simulink model "coif1_7_Level"  (R2021a)
settings: Solver=VariableStepAuto  StartTime=0.0  StopTime=8  RelTol=1e-3
undefined symbols (not defined in the file): lambda2
libraries: dspsigops x15, dspquant2 x1
(part 1 of 4)
settings Model: Creator=Bhea Vasquez  LastModifiedBy=Bhea Vasquez

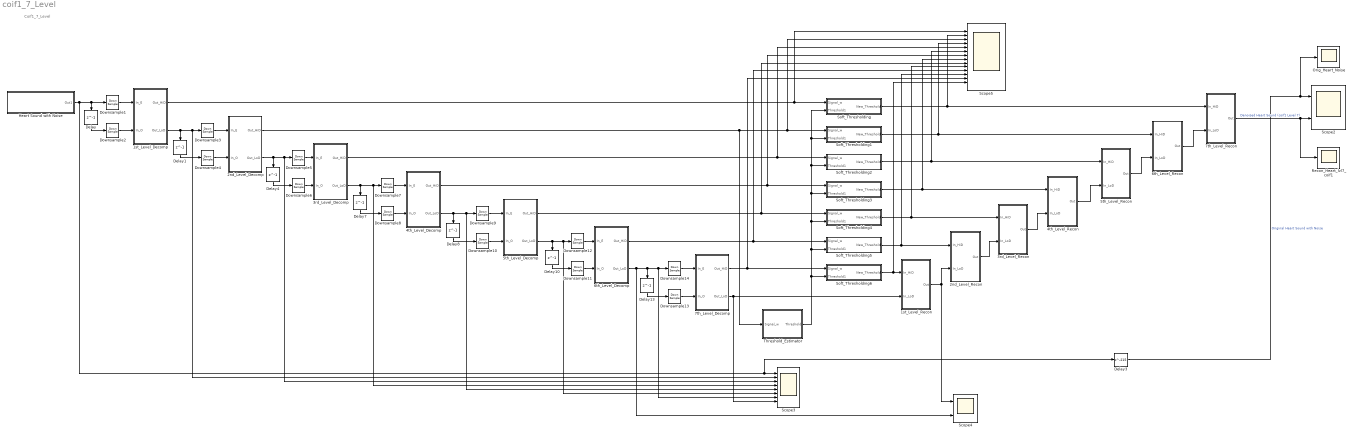
== system coif1_7_Level ==
  note: Coif1_7_Level
  1st_Level_Decomp : Subsystem
  1st_Level_Recon : Subsystem
  2nd_Level_Decomp : Subsystem
  2nd_Level_Recon : Subsystem
  3rd_Level_Decomp : Subsystem
  3rd_Level_Recon : Subsystem
  4th_Level_Decomp : Subsystem
  4th_Level_Recon : Subsystem
  5th_Level_Decomp : Subsystem
  5th_Level_Recon : Subsystem
  6th_Level_Decomp : Subsystem
  6th_Level_Recon : Subsystem
  7th_Level_Decomp : Subsystem
  7th_Level_Recon : Subsystem
  Delay{,1,4,7..8,10,13} (7 alike) : Delay  DelayLength=1  SampleTime=1/44100
  Delay3 : Delay  DelayLength=215  SampleTime=1/44100
  Downsample{1..14} (14 alike) : DownSample  N=30
  Heart Sound with Noise : Subsystem
  Orig_Heart_Noise : Scope
  Recon_Heart_lvl7_coif1 : Scope
  Scope2 : Scope  NumInputPorts=2
  Scope3 : Scope  NumInputPorts=8
  Scope4 : Scope  NumInputPorts=2
  Scope5 : Scope  NumInputPorts=14
  Soft_Thresholding : Subsystem
  Soft_Thresholding1 : Subsystem
  Soft_Thresholding2 : Subsystem
  Soft_Thresholding3 : Subsystem
  Soft_Thresholding4 : Subsystem
  Soft_Thresholding5 : Subsystem
  Soft_Thresholding6 : Subsystem
  Threshold_Estimator : Subsystem
  wires:
  5th_Level_Decomp/2(Out_LoD) -> Scope3/6, Downsample12/1, Delay10/1
  Downsample11/1 -> 6th_Level_Decomp/2(In_O)
  Delay10/1 -> Downsample11/1
  Downsample12/1 -> 6th_Level_Decomp/1(In_E)
  4th_Level_Decomp/2(Out_LoD) -> Scope3/5, Downsample9/1, Delay8/1
  Delay4/1 -> Downsample6/1
  1st_Level_Decomp/2(Out_LoD) -> Scope3/2, Downsample3/1, Delay1/1
  Downsample9/1 -> 5th_Level_Decomp/1(In_E)
  Downsample3/1 -> 2nd_Level_Decomp/1(In_E)
  Heart Sound with Noise/1(Out1) -> Delay3/1, Scope3/1, Downsample1/1, Delay/1
  Downsample6/1 -> 3rd_Level_Decomp/2(In_O)
  Delay7/1 -> Downsample8/1
  Downsample8/1 -> 4th_Level_Decomp/2(In_O)
  Downsample1/1 -> 1st_Level_Decomp/1(In_E)
  Downsample5/1 -> 3rd_Level_Decomp/1(In_E)
  Delay8/1 -> Downsample10/1
  Downsample7/1 -> 4th_Level_Decomp/1(In_E)
  Downsample4/1 -> 2nd_Level_Decomp/2(In_O)
  Delay1/1 -> Downsample4/1
  2nd_Level_Decomp/2(Out_LoD) -> Scope3/3, Downsample5/1, Delay4/1
  Downsample2/1 -> 1st_Level_Decomp/2(In_O)
  3rd_Level_Decomp/2(Out_LoD) -> Scope3/4, Downsample7/1, Delay7/1
  Downsample10/1 -> 5th_Level_Decomp/2(In_O)
  Downsample13/1 -> 7th_Level_Decomp/2(In_O)
  Downsample14/1 -> 7th_Level_Decomp/1(In_E)
  Delay13/1 -> Downsample13/1
  6th_Level_Decomp/2(Out_LoD) -> Scope4/2, Scope3/7, Downsample14/1, Delay13/1
  Threshold_Estimator/1(Threshold) -> Soft_Thresholding6/2(Threshold1), Soft_Thresholding5/2(Threshold1), Soft_Thresholding4/2(Threshold1), Soft_Thresholding3/2(Threshold1), Soft_Thresholding2/2(Threshold1), Soft_Thresholding1/2(Threshold1), Soft_Thresholding/2(Threshold1)
  4th_Level_Decomp/1(Out_HiD) -> Soft_Thresholding3/1(Signal_w), Scope5/7
  5th_Level_Decomp/1(Out_HiD) -> Scope5/9, Soft_Thresholding4/1(Signal_w)
  3rd_Level_Decomp/1(Out_HiD) -> Scope5/5, Soft_Thresholding2/1(Signal_w)
  2nd_Level_Decomp/1(Out_HiD) -> Threshold_Estimator/1(Signal_w), Scope5/3, Soft_Thresholding1/1(Signal_w)
  6th_Level_Decomp/1(Out_HiD) -> Scope5/11, Soft_Thresholding5/1(Signal_w)
  1st_Level_Decomp/1(Out_HiD) -> Scope5/1, Soft_Thresholding/1(Signal_w)
  7th_Level_Decomp/1(Out_HiD) -> Scope5/13, Soft_Thresholding6/1(Signal_w)
  7th_Level_Decomp/2(Out_LoD) -> Scope3/8, 1st_Level_Recon/2(In_LoD)
  Soft_Thresholding6/1(New_Threshold) -> Scope5/14, 1st_Level_Recon/1(In_HiD)
  Soft_Thresholding/1(New_Threshold) -> 7th_Level_Recon/1(In_HiD), Scope5/2
  Soft_Thresholding1/1(New_Threshold) -> 6th_Level_Recon/1(In_HiD), Scope5/4
  6th_Level_Recon/1(Out) -> 7th_Level_Recon/2(In_LoD)
  Soft_Thresholding2/1(New_Threshold) -> 5th_Level_Recon/1(In_HiD), Scope5/6
  Soft_Thresholding3/1(New_Threshold) -> 4th_Level_Recon/1(In_HiD), Scope5/8
  Soft_Thresholding4/1(New_Threshold) -> 3rd_Level_Recon/1(In_HiD), Scope5/10
  Soft_Thresholding5/1(New_Threshold) -> 2nd_Level_Recon/1(In_HiD), Scope5/12
  Delay/1 -> Downsample2/1
  7th_Level_Recon/1(Out) -> Scope2/2, Recon_Heart_lvl7_coif1/1  "Denoised Heart Sound (coif1 Level 7)"
  1st_Level_Recon/1(Out) -> Scope4/1, 2nd_Level_Recon/2(In_LoD)
  4th_Level_Recon/1(Out) -> 5th_Level_Recon/2(In_LoD)
  Delay3/1 -> Scope2/1, Orig_Heart_Noise/1  "Original Heart Sound with Noise"
  2nd_Level_Recon/1(Out) -> 3rd_Level_Recon/2(In_LoD)
  3rd_Level_Recon/1(Out) -> 4th_Level_Recon/2(In_LoD)
  5th_Level_Recon/1(Out) -> 6th_Level_Recon/2(In_LoD)

== system coif1_7_Level/1st_Level_Decomp ==
  In_E : Inport  OutDataTypeStr=double  SampleTime=1/44100
  In_O : Inport  Port=2  OutDataTypeStr=double  SampleTime=1/44100
  Add : Sum  AccumDataTypeStr=double  OutDataTypeStr=double  LockScale=on
  Add1 : Sum  AccumDataTypeStr=double  OutDataTypeStr=double  LockScale=on
  Delay1 : Delay  DelayLength=1  SampleTime=1/44100
  Delay2 : Delay  DelayLength=1  SampleTime=1/44100
  Divide1 : Product  Inputs=*/  OutDataTypeStr=double
  Divide2 : Product  Inputs=*/  OutDataTypeStr=double
  HiD : Constant  Value=0.99803726+0.738418237  OutDataTypeStr=double  SampleTime=1/44100
  HiD_Even : Subsystem
  HiD_Odd : Subsystem
  LoD : Constant  Value=0.738418237+0.99803726  OutDataTypeStr=double  SampleTime=1/44100
  LoD_Even : Subsystem
  LoD_Odd : Subsystem
  Out_HiD : Outport  OutDataTypeStr=double  SampleTime=1/44100
  Out_LoD : Outport  Port=2  OutDataTypeStr=double  SampleTime=1/44100
  wires:
  HiD_Even/1(Out_HiD_e) -> Add/1
  HiD_Odd/1(Out_HiD_o) -> Add/2
  LoD_Even/1(Out_LoD_e) -> Add1/1
  Delay1/1 -> Out_HiD/1
  Delay2/1 -> Out_LoD/1
  In_E/1 -> LoD_Even/1(In_LoD_e), HiD_Even/1(In_HiD_e)
  In_O/1 -> HiD_Odd/1(In_HiD_o), LoD_Odd/1(In_LoD_o)
  Add/1 -> Divide1/1
  Add1/1 -> Divide2/1
  LoD_Odd/1(Out_LoD_o) -> Add1/2
  LoD/1 -> Divide2/2
  Divide2/1 -> Delay2/1
  HiD/1 -> Divide1/2
  Divide1/1 -> Delay1/1

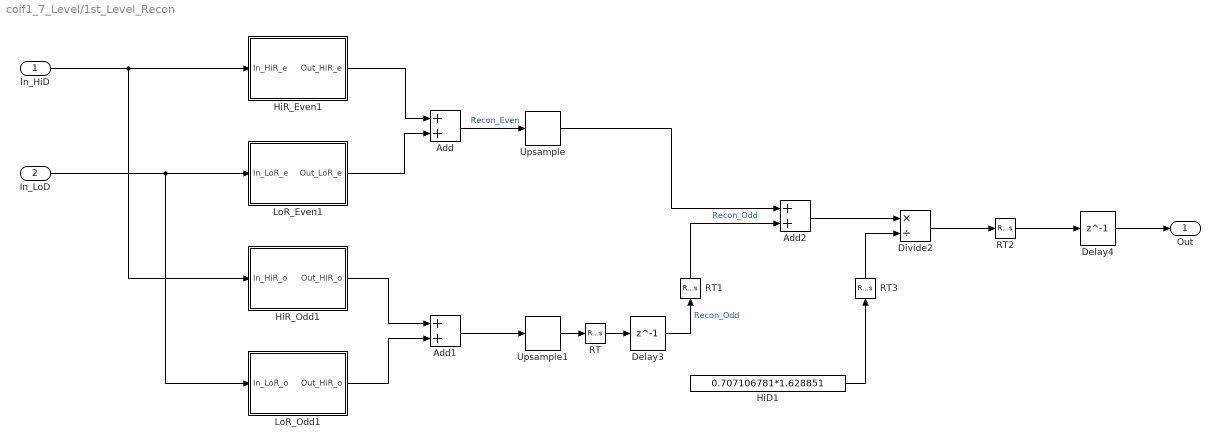
== system coif1_7_Level/1st_Level_Recon ==
  In_HiD : Inport  OutDataTypeStr=double  SampleTime=1/44100
  In_LoD : Inport  Port=2  OutDataTypeStr=double  SampleTime=1/44100
  Add : Sum  AccumDataTypeStr=double  OutDataTypeStr=double
  Add1 : Sum  AccumDataTypeStr=double  OutDataTypeStr=double
  Add2 : Sum  AccumDataTypeStr=double  OutDataTypeStr=double
  Delay3 : Delay  DelayLength=1  SampleTime=1/44100
  Delay4 : Delay  DelayLength=1  SampleTime=1/44100
  Divide2 : Product  Inputs=*/  OutDataTypeStr=double  RndMeth=Zero  SaturateOnIntegerOverflow=on
  HiD1 : Constant  Value=0.707106781*1.628851  OutDataTypeStr=double  SampleTime=1/44100
  HiR_Even1 : Subsystem
  HiR_Odd1 : Subsystem
  LoR_Even1 : Subsystem
  LoR_Odd1 : Subsystem
  RT : RateTransition  OutPortSampleTime=2.267573696145125e-05
  RT1 : RateTransition  OutPortSampleTime=1.133786848072562e-05
  RT2 : RateTransition  OutPortSampleTime=2.267573696145125e-05
  RT3 : RateTransition  OutPortSampleTime=1.133786848072562e-05
  Upsample : dspsigops/Upsample  N=30  phase=0  RateOptions=Allow multirate processing  ic=0  mode=Unused parameter value
  Upsample1 : dspsigops/Upsample  N=30  phase=0  RateOptions=Allow multirate processing  ic=0  mode=Unused parameter value
  Out : Outport  OutDataTypeStr=double  SampleTime=1/44100
  wires:
  LoR_Odd1/1(Out_HiR_o) -> Add1/2
  HiR_Even1/1(Out_HiR_e) -> Add/1
  HiR_Odd1/1(Out_HiR_o) -> Add1/1
  In_HiD/1 -> HiR_Odd1/1(In_HiR_o), HiR_Even1/1(In_HiR_e)
  LoR_Even1/1(Out_LoR_e) -> Add/2
  In_LoD/1 -> LoR_Odd1/1(In_LoR_o), LoR_Even1/1(In_LoR_e)
  Add2/1 -> Divide2/1
  Upsample1/1 -> RT/1
  Delay3/1 -> RT1/1  "Recon_Odd"
  Add1/1 -> Upsample1/1
  Divide2/1 -> RT2/1
  Add/1 -> Upsample/1  "Recon_Even"
  Upsample/1 -> Add2/1
  RT2/1 -> Delay4/1
  RT1/1 -> Add2/2  "Recon_Odd"
  Delay4/1 -> Out/1
  RT/1 -> Delay3/1
  RT3/1 -> Divide2/2
  HiD1/1 -> RT3/1

== system coif1_7_Level/2nd_Level_Decomp ==
  In_E : Inport  OutDataTypeStr=double  SampleTime=1/44100
  In_O : Inport  Port=2  OutDataTypeStr=double  SampleTime=1/44100
  Add : Sum  AccumDataTypeStr=double  OutDataTypeStr=double  LockScale=on
  Add1 : Sum  AccumDataTypeStr=double  OutDataTypeStr=double  LockScale=on
  Delay1 : Delay  DelayLength=1  SampleTime=1/44100
  Delay2 : Delay  DelayLength=1  SampleTime=1/44100
  Divide1 : Product  Inputs=*/  OutDataTypeStr=double
  Divide2 : Product  Inputs=*/  OutDataTypeStr=double
  HiD : Constant  Value=0.99803726+0.738418237  OutDataTypeStr=double  SampleTime=1/44100
  HiD_Even : Subsystem
  HiD_Odd : Subsystem
  LoD : Constant  Value=0.738418237+0.99803726  OutDataTypeStr=double  SampleTime=1/44100
  LoD_Even : Subsystem
  LoD_Odd : Subsystem
  Out_HiD : Outport  OutDataTypeStr=double  SampleTime=1/44100
  Out_LoD : Outport  Port=2  OutDataTypeStr=double  SampleTime=1/44100
  wires:
  HiD_Even/1(Out_HiD_e) -> Add/1
  HiD_Odd/1(Out_HiD_o) -> Add/2
  LoD_Even/1(Out_LoD_e) -> Add1/1
  Delay1/1 -> Out_HiD/1
  Delay2/1 -> Out_LoD/1
  In_E/1 -> LoD_Even/1(In_LoD_e), HiD_Even/1(In_HiD_e)
  In_O/1 -> HiD_Odd/1(In_HiD_o), LoD_Odd/1(In_LoD_o)
  Add/1 -> Divide1/1
  Add1/1 -> Divide2/1
  LoD_Odd/1(Out_LoD_o) -> Add1/2
  LoD/1 -> Divide2/2
  Divide2/1 -> Delay2/1
  HiD/1 -> Divide1/2
  Divide1/1 -> Delay1/1

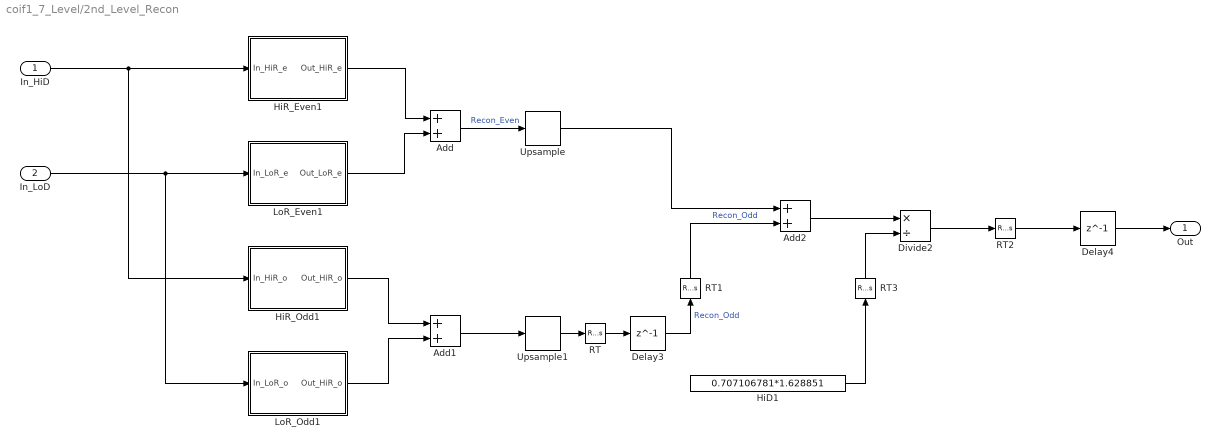
== system coif1_7_Level/2nd_Level_Recon ==
  In_HiD : Inport  OutDataTypeStr=double  SampleTime=1/44100
  In_LoD : Inport  Port=2  OutDataTypeStr=double  SampleTime=1/44100
  Add : Sum  AccumDataTypeStr=double  OutDataTypeStr=double
  Add1 : Sum  AccumDataTypeStr=double  OutDataTypeStr=double
  Add2 : Sum  AccumDataTypeStr=double  OutDataTypeStr=double
  Delay3 : Delay  DelayLength=1  SampleTime=1/44100
  Delay4 : Delay  DelayLength=1  SampleTime=1/44100
  Divide2 : Product  Inputs=*/  OutDataTypeStr=double  RndMeth=Zero  SaturateOnIntegerOverflow=on
  HiD1 : Constant  Value=0.707106781*1.628851  OutDataTypeStr=double  SampleTime=1/44100
  HiR_Even1 : Subsystem
  HiR_Odd1 : Subsystem
  LoR_Even1 : Subsystem
  LoR_Odd1 : Subsystem
  RT : RateTransition  OutPortSampleTime=2.267573696145125e-05
  RT1 : RateTransition  OutPortSampleTime=1.133786848072562e-05
  RT2 : RateTransition  OutPortSampleTime=2.267573696145125e-05
  RT3 : RateTransition  OutPortSampleTime=1.133786848072562e-05
  Upsample : dspsigops/Upsample  N=30  phase=0  RateOptions=Allow multirate processing  ic=0  mode=Unused parameter value
  Upsample1 : dspsigops/Upsample  N=30  phase=0  RateOptions=Allow multirate processing  ic=0  mode=Unused parameter value
  Out : Outport  OutDataTypeStr=double  SampleTime=1/44100
  wires:
  LoR_Odd1/1(Out_HiR_o) -> Add1/2
  HiR_Even1/1(Out_HiR_e) -> Add/1
  HiR_Odd1/1(Out_HiR_o) -> Add1/1
  In_HiD/1 -> HiR_Odd1/1(In_HiR_o), HiR_Even1/1(In_HiR_e)
  LoR_Even1/1(Out_LoR_e) -> Add/2
  In_LoD/1 -> LoR_Odd1/1(In_LoR_o), LoR_Even1/1(In_LoR_e)
  Add2/1 -> Divide2/1
  Upsample1/1 -> RT/1
  Delay3/1 -> RT1/1  "Recon_Odd"
  Add1/1 -> Upsample1/1
  Divide2/1 -> RT2/1
  Add/1 -> Upsample/1  "Recon_Even"
  Upsample/1 -> Add2/1
  RT2/1 -> Delay4/1
  RT1/1 -> Add2/2  "Recon_Odd"
  Delay4/1 -> Out/1
  RT/1 -> Delay3/1
  RT3/1 -> Divide2/2
  HiD1/1 -> RT3/1

== system coif1_7_Level/3rd_Level_Decomp ==
  In_E : Inport  OutDataTypeStr=double  SampleTime=1/44100
  In_O : Inport  Port=2  OutDataTypeStr=double  SampleTime=1/44100
  Add : Sum  AccumDataTypeStr=double  OutDataTypeStr=double  LockScale=on
  Add1 : Sum  AccumDataTypeStr=double  OutDataTypeStr=double  LockScale=on
  Delay1 : Delay  DelayLength=1  SampleTime=1/44100
  Delay2 : Delay  DelayLength=1  SampleTime=1/44100
  Divide1 : Product  Inputs=*/  OutDataTypeStr=double
  Divide2 : Product  Inputs=*/  OutDataTypeStr=double
  HiD : Constant  Value=0.99803726+0.738418237  OutDataTypeStr=double  SampleTime=1/44100
  HiD_Even : Subsystem
  HiD_Odd : Subsystem
  LoD : Constant  Value=0.738418237+0.99803726  OutDataTypeStr=double  SampleTime=1/44100
  LoD_Even : Subsystem
  LoD_Odd : Subsystem
  Out_HiD : Outport  OutDataTypeStr=double  SampleTime=1/44100
  Out_LoD : Outport  Port=2  OutDataTypeStr=double  SampleTime=1/44100
  wires:
  HiD_Even/1(Out_HiD_e) -> Add/1
  HiD_Odd/1(Out_HiD_o) -> Add/2
  LoD_Even/1(Out_LoD_e) -> Add1/1
  Delay1/1 -> Out_HiD/1
  Delay2/1 -> Out_LoD/1
  In_E/1 -> LoD_Even/1(In_LoD_e), HiD_Even/1(In_HiD_e)
  In_O/1 -> HiD_Odd/1(In_HiD_o), LoD_Odd/1(In_LoD_o)
  Add/1 -> Divide1/1
  Add1/1 -> Divide2/1
  LoD_Odd/1(Out_LoD_o) -> Add1/2
  LoD/1 -> Divide2/2
  Divide2/1 -> Delay2/1
  HiD/1 -> Divide1/2
  Divide1/1 -> Delay1/1

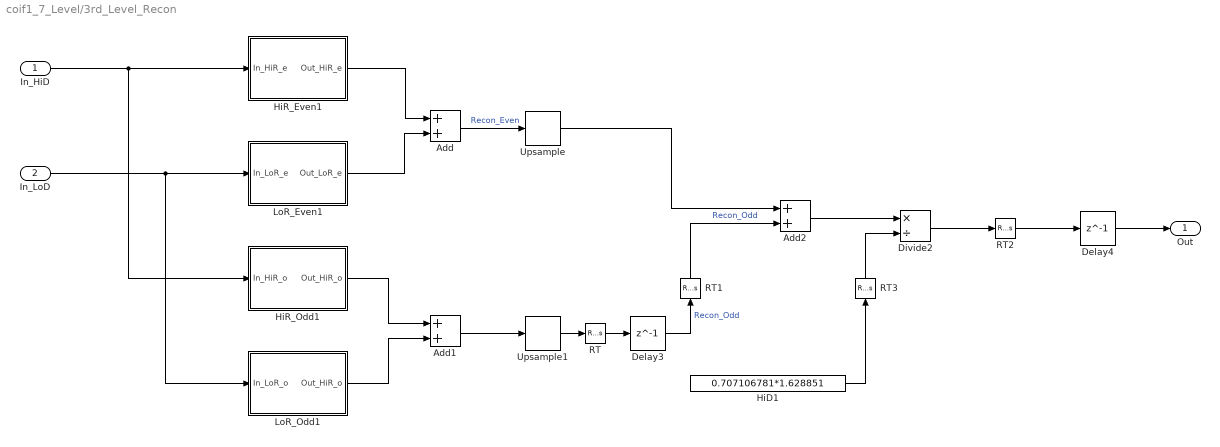
== system coif1_7_Level/3rd_Level_Recon ==
  In_HiD : Inport  OutDataTypeStr=double  SampleTime=1/44100
  In_LoD : Inport  Port=2  OutDataTypeStr=double  SampleTime=1/44100
  Add : Sum  AccumDataTypeStr=double  OutDataTypeStr=double
  Add1 : Sum  AccumDataTypeStr=double  OutDataTypeStr=double
  Add2 : Sum  AccumDataTypeStr=double  OutDataTypeStr=double
  Delay3 : Delay  DelayLength=1  SampleTime=1/44100
  Delay4 : Delay  DelayLength=1  SampleTime=1/44100
  Divide2 : Product  Inputs=*/  OutDataTypeStr=double  RndMeth=Zero  SaturateOnIntegerOverflow=on
  HiD1 : Constant  Value=0.707106781*1.628851  OutDataTypeStr=double  SampleTime=1/44100
  HiR_Even1 : Subsystem
  HiR_Odd1 : Subsystem
  LoR_Even1 : Subsystem
  LoR_Odd1 : Subsystem
  RT : RateTransition  OutPortSampleTime=2.267573696145125e-05
  RT1 : RateTransition  OutPortSampleTime=1.133786848072562e-05
  RT2 : RateTransition  OutPortSampleTime=2.267573696145125e-05
  RT3 : RateTransition  OutPortSampleTime=1.133786848072562e-05
  Upsample : dspsigops/Upsample  N=30  phase=0  RateOptions=Allow multirate processing  ic=0  mode=Unused parameter value
  Upsample1 : dspsigops/Upsample  N=30  phase=0  RateOptions=Allow multirate processing  ic=0  mode=Unused parameter value
  Out : Outport  OutDataTypeStr=double  SampleTime=1/44100
  wires:
  LoR_Odd1/1(Out_HiR_o) -> Add1/2
  HiR_Even1/1(Out_HiR_e) -> Add/1
  HiR_Odd1/1(Out_HiR_o) -> Add1/1
  In_HiD/1 -> HiR_Odd1/1(In_HiR_o), HiR_Even1/1(In_HiR_e)
  LoR_Even1/1(Out_LoR_e) -> Add/2
  In_LoD/1 -> LoR_Odd1/1(In_LoR_o), LoR_Even1/1(In_LoR_e)
  Add2/1 -> Divide2/1
  Upsample1/1 -> RT/1
  Delay3/1 -> RT1/1  "Recon_Odd"
  Add1/1 -> Upsample1/1
  Divide2/1 -> RT2/1
  Add/1 -> Upsample/1  "Recon_Even"
  Upsample/1 -> Add2/1
  RT2/1 -> Delay4/1
  RT1/1 -> Add2/2  "Recon_Odd"
  Delay4/1 -> Out/1
  RT/1 -> Delay3/1
  RT3/1 -> Divide2/2
  HiD1/1 -> RT3/1

== system coif1_7_Level/4th_Level_Decomp ==
  In_E : Inport  OutDataTypeStr=double  SampleTime=1/44100
  In_O : Inport  Port=2  OutDataTypeStr=double  SampleTime=1/44100
  Add : Sum  AccumDataTypeStr=double  OutDataTypeStr=double  LockScale=on
  Add1 : Sum  AccumDataTypeStr=double  OutDataTypeStr=double  LockScale=on
  Delay1 : Delay  DelayLength=1  SampleTime=1/44100
  Delay2 : Delay  DelayLength=1  SampleTime=1/44100
  Divide1 : Product  Inputs=*/  OutDataTypeStr=double
  Divide2 : Product  Inputs=*/  OutDataTypeStr=double
  HiD : Constant  Value=0.99803726+0.738418237  OutDataTypeStr=double  SampleTime=1/44100
  HiD_Even : Subsystem
  HiD_Odd : Subsystem
  LoD : Constant  Value=0.738418237+0.99803726  OutDataTypeStr=double  SampleTime=1/44100
  LoD_Even : Subsystem
  LoD_Odd : Subsystem
  Out_HiD : Outport  OutDataTypeStr=double  SampleTime=1/44100
  Out_LoD : Outport  Port=2  OutDataTypeStr=double  SampleTime=1/44100
  wires:
  HiD_Even/1(Out_HiD_e) -> Add/1
  HiD_Odd/1(Out_HiD_o) -> Add/2
  LoD_Even/1(Out_LoD_e) -> Add1/1
  Delay1/1 -> Out_HiD/1
  Delay2/1 -> Out_LoD/1
  In_E/1 -> LoD_Even/1(In_LoD_e), HiD_Even/1(In_HiD_e)
  In_O/1 -> HiD_Odd/1(In_HiD_o), LoD_Odd/1(In_LoD_o)
  Add/1 -> Divide1/1
  Add1/1 -> Divide2/1
  LoD_Odd/1(Out_LoD_o) -> Add1/2
  LoD/1 -> Divide2/2
  Divide2/1 -> Delay2/1
  HiD/1 -> Divide1/2
  Divide1/1 -> Delay1/1

== system coif1_7_Level/4th_Level_Recon ==
  In_HiD : Inport  OutDataTypeStr=double  SampleTime=1/44100
  In_LoD : Inport  Port=2  OutDataTypeStr=double  SampleTime=1/44100
  Add : Sum  AccumDataTypeStr=double  OutDataTypeStr=double
  Add1 : Sum  AccumDataTypeStr=double  OutDataTypeStr=double
  Add2 : Sum  AccumDataTypeStr=double  OutDataTypeStr=double
  Delay3 : Delay  DelayLength=1  SampleTime=1/44100
  Delay4 : Delay  DelayLength=1  SampleTime=1/44100
  Divide2 : Product  Inputs=*/  OutDataTypeStr=double  RndMeth=Zero  SaturateOnIntegerOverflow=on
  HiD1 : Constant  Value=0.707106781*1.628851  OutDataTypeStr=double  SampleTime=1/44100
  HiR_Even1 : Subsystem
  HiR_Odd1 : Subsystem
  LoR_Even1 : Subsystem
  LoR_Odd1 : Subsystem
  RT : RateTransition  OutPortSampleTime=2.267573696145125e-05
  RT1 : RateTransition  OutPortSampleTime=1.133786848072562e-05
  RT2 : RateTransition  OutPortSampleTime=2.267573696145125e-05
  RT3 : RateTransition  OutPortSampleTime=1.133786848072562e-05
  Upsample : dspsigops/Upsample  N=30  phase=0  RateOptions=Allow multirate processing  ic=0  mode=Unused parameter value
  Upsample1 : dspsigops/Upsample  N=30  phase=0  RateOptions=Allow multirate processing  ic=0  mode=Unused parameter value
  Out : Outport  OutDataTypeStr=double  SampleTime=1/44100
  wires:
  LoR_Odd1/1(Out_HiR_o) -> Add1/2
  HiR_Even1/1(Out_HiR_e) -> Add/1
  HiR_Odd1/1(Out_HiR_o) -> Add1/1
  In_HiD/1 -> HiR_Odd1/1(In_HiR_o), HiR_Even1/1(In_HiR_e)
  LoR_Even1/1(Out_LoR_e) -> Add/2
  In_LoD/1 -> LoR_Odd1/1(In_LoR_o), LoR_Even1/1(In_LoR_e)
  Add2/1 -> Divide2/1
  Upsample1/1 -> RT/1
  Delay3/1 -> RT1/1  "Recon_Odd"
  Add1/1 -> Upsample1/1
  Divide2/1 -> RT2/1
  Add/1 -> Upsample/1  "Recon_Even"
  Upsample/1 -> Add2/1
  RT2/1 -> Delay4/1
  RT1/1 -> Add2/2  "Recon_Odd"
  Delay4/1 -> Out/1
  RT/1 -> Delay3/1
  RT3/1 -> Divide2/2
  HiD1/1 -> RT3/1

== system coif1_7_Level/5th_Level_Decomp ==
  In_E : Inport  OutDataTypeStr=double  SampleTime=1/44100
  In_O : Inport  Port=2  OutDataTypeStr=double  SampleTime=1/44100
  Add : Sum  AccumDataTypeStr=double  OutDataTypeStr=double  LockScale=on
  Add1 : Sum  AccumDataTypeStr=double  OutDataTypeStr=double  LockScale=on
  Delay1 : Delay  DelayLength=1  SampleTime=1/44100
  Delay2 : Delay  DelayLength=1  SampleTime=1/44100
  Divide1 : Product  Inputs=*/  OutDataTypeStr=double
  Divide2 : Product  Inputs=*/  OutDataTypeStr=double
  HiD : Constant  Value=0.99803726+0.738418237  OutDataTypeStr=double  SampleTime=1/44100
  HiD_Even : Subsystem
  HiD_Odd : Subsystem
  LoD : Constant  Value=0.738418237+0.99803726  OutDataTypeStr=double  SampleTime=1/44100
  LoD_Even : Subsystem
  LoD_Odd : Subsystem
  Out_HiD : Outport  OutDataTypeStr=double  SampleTime=1/44100
  Out_LoD : Outport  Port=2  OutDataTypeStr=double  SampleTime=1/44100
  wires:
  HiD_Even/1(Out_HiD_e) -> Add/1
  HiD_Odd/1(Out_HiD_o) -> Add/2
  LoD_Even/1(Out_LoD_e) -> Add1/1
  Delay1/1 -> Out_HiD/1
  Delay2/1 -> Out_LoD/1
  In_E/1 -> LoD_Even/1(In_LoD_e), HiD_Even/1(In_HiD_e)
  In_O/1 -> HiD_Odd/1(In_HiD_o), LoD_Odd/1(In_LoD_o)
  Add/1 -> Divide1/1
  Add1/1 -> Divide2/1
  LoD_Odd/1(Out_LoD_o) -> Add1/2
  LoD/1 -> Divide2/2
  Divide2/1 -> Delay2/1
  HiD/1 -> Divide1/2
  Divide1/1 -> Delay1/1

== system coif1_7_Level/5th_Level_Recon ==
  In_HiD : Inport  OutDataTypeStr=double  SampleTime=1/44100
  In_LoD : Inport  Port=2  OutDataTypeStr=double  SampleTime=1/44100
  Add : Sum  AccumDataTypeStr=double  OutDataTypeStr=double
  Add1 : Sum  AccumDataTypeStr=double  OutDataTypeStr=double
  Add2 : Sum  AccumDataTypeStr=double  OutDataTypeStr=double
  Delay3 : Delay  DelayLength=1  SampleTime=1/44100
  Delay4 : Delay  DelayLength=1  SampleTime=1/44100
  Divide2 : Product  Inputs=*/  OutDataTypeStr=double  RndMeth=Zero  SaturateOnIntegerOverflow=on
  HiD1 : Constant  Value=0.707106781*1.628851  OutDataTypeStr=double  SampleTime=1/44100
  HiR_Even1 : Subsystem
  HiR_Odd1 : Subsystem
  LoR_Even1 : Subsystem
  LoR_Odd1 : Subsystem
  RT : RateTransition  OutPortSampleTime=2.267573696145125e-05
  RT1 : RateTransition  OutPortSampleTime=1.133786848072562e-05
  RT2 : RateTransition  OutPortSampleTime=2.267573696145125e-05
  RT3 : RateTransition  OutPortSampleTime=1.133786848072562e-05
  Upsample : dspsigops/Upsample  N=30  phase=0  RateOptions=Allow multirate processing  ic=0  mode=Unused parameter value
  Upsample1 : dspsigops/Upsample  N=30  phase=0  RateOptions=Allow multirate processing  ic=0  mode=Unused parameter value
  Out : Outport  OutDataTypeStr=double  SampleTime=1/44100
  wires:
  LoR_Odd1/1(Out_HiR_o) -> Add1/2
  HiR_Even1/1(Out_HiR_e) -> Add/1
  HiR_Odd1/1(Out_HiR_o) -> Add1/1
  In_HiD/1 -> HiR_Odd1/1(In_HiR_o), HiR_Even1/1(In_HiR_e)
  LoR_Even1/1(Out_LoR_e) -> Add/2
  In_LoD/1 -> LoR_Odd1/1(In_LoR_o), LoR_Even1/1(In_LoR_e)
  Add2/1 -> Divide2/1
  Upsample1/1 -> RT/1
  Delay3/1 -> RT1/1  "Recon_Odd"
  Add1/1 -> Upsample1/1
  Divide2/1 -> RT2/1
  Add/1 -> Upsample/1  "Recon_Even"
  Upsample/1 -> Add2/1
  RT2/1 -> Delay4/1
  RT1/1 -> Add2/2  "Recon_Odd"
  Delay4/1 -> Out/1
  RT/1 -> Delay3/1
  RT3/1 -> Divide2/2
  HiD1/1 -> RT3/1

== system coif1_7_Level/6th_Level_Decomp ==
  In_E : Inport  OutDataTypeStr=double  SampleTime=1/44100
  In_O : Inport  Port=2  OutDataTypeStr=double  SampleTime=1/44100
  Add : Sum  AccumDataTypeStr=double  OutDataTypeStr=double  LockScale=on
  Add1 : Sum  AccumDataTypeStr=double  OutDataTypeStr=double  LockScale=on
  Delay1 : Delay  DelayLength=1  SampleTime=1/44100
  Delay2 : Delay  DelayLength=1  SampleTime=1/44100
  Divide1 : Product  Inputs=*/  OutDataTypeStr=double
  Divide2 : Product  Inputs=*/  OutDataTypeStr=double
  HiD : Constant  Value=0.99803726+0.738418237  OutDataTypeStr=double  SampleTime=1/44100
  HiD_Even : Subsystem
  HiD_Odd : Subsystem
  LoD : Constant  Value=0.738418237+0.99803726  OutDataTypeStr=double  SampleTime=1/44100
  LoD_Even : Subsystem
  LoD_Odd : Subsystem
  Out_HiD : Outport  OutDataTypeStr=double  SampleTime=1/44100
  Out_LoD : Outport  Port=2  OutDataTypeStr=double  SampleTime=1/44100
  wires:
  HiD_Even/1(Out_HiD_e) -> Add/1
  HiD_Odd/1(Out_HiD_o) -> Add/2
  LoD_Even/1(Out_LoD_e) -> Add1/1
  Delay1/1 -> Out_HiD/1
  Delay2/1 -> Out_LoD/1
  In_E/1 -> LoD_Even/1(In_LoD_e), HiD_Even/1(In_HiD_e)
  In_O/1 -> HiD_Odd/1(In_HiD_o), LoD_Odd/1(In_LoD_o)
  Add/1 -> Divide1/1
  Add1/1 -> Divide2/1
  LoD_Odd/1(Out_LoD_o) -> Add1/2
  LoD/1 -> Divide2/2
  Divide2/1 -> Delay2/1
  HiD/1 -> Divide1/2
  Divide1/1 -> Delay1/1

== system coif1_7_Level/6th_Level_Recon ==
  In_HiD : Inport  OutDataTypeStr=double  SampleTime=1/44100
  In_LoD : Inport  Port=2  OutDataTypeStr=double  SampleTime=1/44100
  Add : Sum  AccumDataTypeStr=double  OutDataTypeStr=double
  Add1 : Sum  AccumDataTypeStr=double  OutDataTypeStr=double
  Add2 : Sum  AccumDataTypeStr=double  OutDataTypeStr=double
  Delay3 : Delay  DelayLength=1  SampleTime=1/44100
  Delay4 : Delay  DelayLength=1  SampleTime=1/44100
  Divide2 : Product  Inputs=*/  OutDataTypeStr=double  RndMeth=Zero  SaturateOnIntegerOverflow=on
  HiD1 : Constant  Value=0.707106781*1.628851  OutDataTypeStr=double  SampleTime=1/44100
  HiR_Even1 : Subsystem
  HiR_Odd1 : Subsystem
  LoR_Even1 : Subsystem
  LoR_Odd1 : Subsystem
  RT : RateTransition  OutPortSampleTime=2.267573696145125e-05
  RT1 : RateTransition  OutPortSampleTime=1.133786848072562e-05
  RT2 : RateTransition  OutPortSampleTime=2.267573696145125e-05
  RT3 : RateTransition  OutPortSampleTime=1.133786848072562e-05
  Upsample : dspsigops/Upsample  N=30  phase=0  RateOptions=Allow multirate processing  ic=0  mode=Unused parameter value
  Upsample1 : dspsigops/Upsample  N=30  phase=0  RateOptions=Allow multirate processing  ic=0  mode=Unused parameter value
  Out : Outport  OutDataTypeStr=double  SampleTime=1/44100
  wires:
  LoR_Odd1/1(Out_HiR_o) -> Add1/2
  HiR_Even1/1(Out_HiR_e) -> Add/1
  HiR_Odd1/1(Out_HiR_o) -> Add1/1
  In_HiD/1 -> HiR_Odd1/1(In_HiR_o), HiR_Even1/1(In_HiR_e)
  LoR_Even1/1(Out_LoR_e) -> Add/2
  In_LoD/1 -> LoR_Odd1/1(In_LoR_o), LoR_Even1/1(In_LoR_e)
  Add2/1 -> Divide2/1
  Upsample1/1 -> RT/1
  Delay3/1 -> RT1/1  "Recon_Odd"
  Add1/1 -> Upsample1/1
  Divide2/1 -> RT2/1
  Add/1 -> Upsample/1  "Recon_Even"
  Upsample/1 -> Add2/1
  RT2/1 -> Delay4/1
  RT1/1 -> Add2/2  "Recon_Odd"
  Delay4/1 -> Out/1
  RT/1 -> Delay3/1
  RT3/1 -> Divide2/2
  HiD1/1 -> RT3/1

== system coif1_7_Level/7th_Level_Decomp ==
  In_E : Inport  OutDataTypeStr=double  SampleTime=1/44100
  In_O : Inport  Port=2  OutDataTypeStr=double  SampleTime=1/44100
  Add : Sum  AccumDataTypeStr=double  OutDataTypeStr=double  LockScale=on
  Add1 : Sum  AccumDataTypeStr=double  OutDataTypeStr=double  LockScale=on
  Delay1 : Delay  DelayLength=1  SampleTime=1/44100
  Delay2 : Delay  DelayLength=1  SampleTime=1/44100
  Divide1 : Product  Inputs=*/  OutDataTypeStr=double
  Divide2 : Product  Inputs=*/  OutDataTypeStr=double
  HiD : Constant  Value=0.99803726+0.738418237  OutDataTypeStr=double  SampleTime=1/44100
  HiD_Even : Subsystem
  HiD_Odd : Subsystem
  LoD : Constant  Value=0.738418237+0.99803726  OutDataTypeStr=double  SampleTime=1/44100
  LoD_Even : Subsystem
  LoD_Odd : Subsystem
  Out_HiD : Outport  OutDataTypeStr=double  SampleTime=1/44100
  Out_LoD : Outport  Port=2  OutDataTypeStr=double  SampleTime=1/44100
  wires:
  HiD_Even/1(Out_HiD_e) -> Add/1
  HiD_Odd/1(Out_HiD_o) -> Add/2
  LoD_Even/1(Out_LoD_e) -> Add1/1
  Delay1/1 -> Out_HiD/1
  Delay2/1 -> Out_LoD/1
  In_E/1 -> LoD_Even/1(In_LoD_e), HiD_Even/1(In_HiD_e)
  In_O/1 -> HiD_Odd/1(In_HiD_o), LoD_Odd/1(In_LoD_o)
  Add/1 -> Divide1/1
  Add1/1 -> Divide2/1
  LoD_Odd/1(Out_LoD_o) -> Add1/2
  LoD/1 -> Divide2/2
  Divide2/1 -> Delay2/1
  HiD/1 -> Divide1/2
  Divide1/1 -> Delay1/1

== system coif1_7_Level/7th_Level_Recon ==
  In_HiD : Inport  OutDataTypeStr=double  SampleTime=1/44100
  In_LoD : Inport  Port=2  OutDataTypeStr=double  SampleTime=1/44100
  Add : Sum  AccumDataTypeStr=double  OutDataTypeStr=double
  Add1 : Sum  AccumDataTypeStr=double  OutDataTypeStr=double
  Add2 : Sum  AccumDataTypeStr=double  OutDataTypeStr=double
  Delay3 : Delay  DelayLength=1  SampleTime=1/44100
  Delay4 : Delay  DelayLength=1  SampleTime=1/44100
  Divide2 : Product  Inputs=*/  OutDataTypeStr=double  RndMeth=Zero  SaturateOnIntegerOverflow=on
  HiD1 : Constant  Value=0.707106781*1.628851  OutDataTypeStr=double  SampleTime=1/44100
  HiR_Even1 : Subsystem
  HiR_Odd1 : Subsystem
  LoR_Even1 : Subsystem
  LoR_Odd1 : Subsystem
  RT : RateTransition  OutPortSampleTime=2.267573696145125e-05
  RT1 : RateTransition  OutPortSampleTime=1.133786848072562e-05
  RT2 : RateTransition  OutPortSampleTime=2.267573696145125e-05
  RT3 : RateTransition  OutPortSampleTime=1.133786848072562e-05
  Upsample : dspsigops/Upsample  N=30  phase=0  RateOptions=Allow multirate processing  ic=0  mode=Unused parameter value
  Upsample1 : dspsigops/Upsample  N=30  phase=0  RateOptions=Allow multirate processing  ic=0  mode=Unused parameter value
  Out : Outport  OutDataTypeStr=double  SampleTime=1/44100
  wires:
  LoR_Odd1/1(Out_HiR_o) -> Add1/2
  HiR_Even1/1(Out_HiR_e) -> Add/1
  HiR_Odd1/1(Out_HiR_o) -> Add1/1
  In_HiD/1 -> HiR_Odd1/1(In_HiR_o), HiR_Even1/1(In_HiR_e)
  LoR_Even1/1(Out_LoR_e) -> Add/2
  In_LoD/1 -> LoR_Odd1/1(In_LoR_o), LoR_Even1/1(In_LoR_e)
  Add2/1 -> Divide2/1
  Upsample1/1 -> RT/1
  Delay3/1 -> RT1/1  "Recon_Odd"
  Add1/1 -> Upsample1/1
  Divide2/1 -> RT2/1
  Add/1 -> Upsample/1  "Recon_Even"
  Upsample/1 -> Add2/1
  RT2/1 -> Delay4/1
  RT1/1 -> Add2/2  "Recon_Odd"
  Delay4/1 -> Out/1
  RT/1 -> Delay3/1
  RT3/1 -> Divide2/2
  HiD1/1 -> RT3/1

== system coif1_7_Level/Heart Sound with Noise ==
  Constant : Constant  Value=80000  OutDataTypeStr=double  SampleTime=1/44100
  Divide : Product  Inputs=*/  OutDataTypeStr=double
  From Workspace1 : FromWorkspace  VariableName=Audio_Heart_Noise  OutDataTypeStr=double  SampleTime=1/44100
  Gain2 : Gain  Gain=5  ParamDataTypeStr=double  OutDataTypeStr=double
  Pulse Generator : DiscretePulseGenerator  PulseType=Time based  Period=0.00022675736  PulseWidth=50
  Quantizer : Quantizer  QuantizationInterval=0.1
  Sample and Hold : dspsigops/Sample and Hold  trig=Rising edge  initCond=0  latchinput=off
  Uniform Encoder : dspquant2/Uniform Encoder  peak=2  bits=8  otype=Unsigned integer
  Out1 : Outport  OutDataTypeStr=double  SampleTime=1/44100
  wires:
  Sample and Hold/1 -> Quantizer/1
  Uniform Encoder/1 -> Divide/1
  Quantizer/1 -> Uniform Encoder/1
  Constant/1 -> Divide/2
  From Workspace1/1 -> Gain2/1
  Pulse Generator/1 -> Sample and Hold/Trigger
  Gain2/1 -> Sample and Hold/1
  Divide/1 -> Out1/1

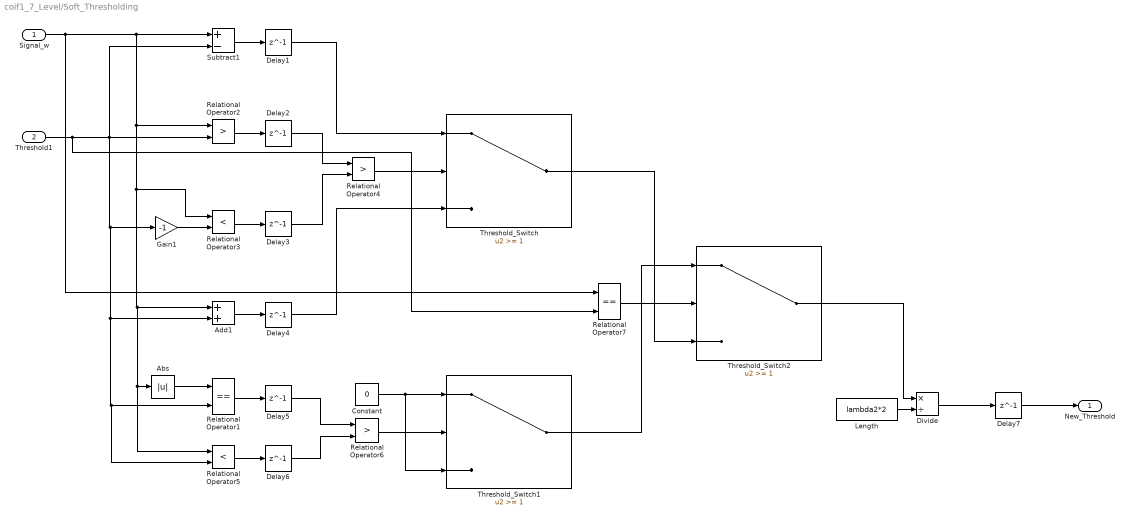
== system coif1_7_Level/Soft_Thresholding ==
  Signal_w : Inport  OutDataTypeStr=double  SampleTime=1/44100
  Threshold1 : Inport  Port=2  OutDataTypeStr=double  SampleTime=1/44100
  Abs : Abs  OutDataTypeStr=double
  Add1 : Sum  AccumDataTypeStr=double  OutDataTypeStr=double
  Constant : Constant  Value=0  OutDataTypeStr=double  SampleTime=1/44100
  Delay{1..7} (7 alike) : Delay  DelayLength=1  SampleTime=1/44100
  Divide : Product  Inputs=*/  OutDataTypeStr=double
  Gain1 : Gain  Gain=-1  ParamDataTypeStr=fixdt(1,16,12)  OutMin=-1  OutMax=-0.99  OutDataTypeStr=double
  Length : Constant  Value=lambda2*2  OutDataTypeStr=double  SampleTime=1/44100
  Relational Operator1 : RelationalOperator  Operator===  OutDataTypeStr=boolean  RndMeth=Simplest
  Relational Operator2 : RelationalOperator  Operator=>  OutDataTypeStr=boolean  RndMeth=Simplest
  Relational Operator3 : RelationalOperator  Operator=<  OutDataTypeStr=boolean  RndMeth=Simplest
  Relational Operator4 : RelationalOperator  Operator=>  OutDataTypeStr=boolean  RndMeth=Simplest
  Relational Operator5 : RelationalOperator  Operator=<  OutDataTypeStr=boolean  RndMeth=Simplest
  Relational Operator6 : RelationalOperator  Operator=>  OutDataTypeStr=boolean  RndMeth=Simplest
  Relational Operator7 : RelationalOperator  Operator===  OutDataTypeStr=boolean  RndMeth=Simplest
  Subtract1 : Sum  Inputs=+-  AccumDataTypeStr=double  OutDataTypeStr=double
  Threshold_Switch : Switch  Threshold=1  OutDataTypeStr=double
  Threshold_Switch1 : Switch  Threshold=1  OutDataTypeStr=double
  Threshold_Switch2 : Switch  Threshold=1  OutDataTypeStr=double
  New_Threshold : Outport  OutDataTypeStr=double  SampleTime=1/44100
  wires:
  Threshold_Switch/1 -> Threshold_Switch2/3
  Relational Operator6/1 -> Threshold_Switch1/2
  Gain1/1 -> Relational Operator3/2
  Delay4/1 -> Threshold_Switch/3
  Add1/1 -> Delay4/1
  Delay2/1 -> Relational Operator4/1
  Delay3/1 -> Relational Operator4/2
  Delay1/1 -> Threshold_Switch/1
  Relational Operator2/1 -> Delay2/1
  Relational Operator3/1 -> Delay3/1
  Relational Operator5/1 -> Delay6/1
  Delay6/1 -> Relational Operator6/2
  Delay5/1 -> Relational Operator6/1
  Threshold1/1 -> Relational Operator2/2, Subtract1/2, Relational Operator5/2, Relational Operator1/2, Add1/2, Gain1/1, Relational Operator7/2
  Abs/1 -> Relational Operator1/1
  Relational Operator4/1 -> Threshold_Switch/2
  Subtract1/1 -> Delay1/1
  Constant/1 -> Threshold_Switch1/3, Threshold_Switch1/1
  Signal_w/1 -> Subtract1/1, Relational Operator2/1, Relational Operator5/1, Abs/1, Add1/1, Relational Operator3/1, Relational Operator7/1
  Relational Operator7/1 -> Threshold_Switch2/2
  Relational Operator1/1 -> Delay5/1
  Threshold_Switch1/1 -> Threshold_Switch2/1
  Threshold_Switch2/1 -> Divide/1
  Length/1 -> Divide/2
  Divide/1 -> Delay7/1
  Delay7/1 -> New_Threshold/1

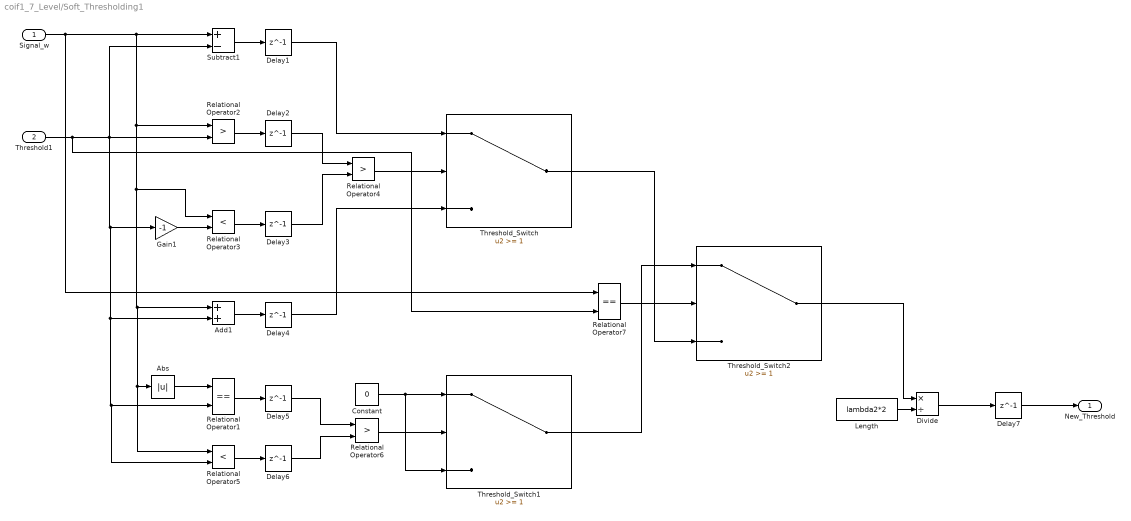
== system coif1_7_Level/Soft_Thresholding1 ==
  Signal_w : Inport  OutDataTypeStr=double  SampleTime=1/44100
  Threshold1 : Inport  Port=2  OutDataTypeStr=double  SampleTime=1/44100
  Abs : Abs  OutDataTypeStr=double
  Add1 : Sum  AccumDataTypeStr=double  OutDataTypeStr=double
  Constant : Constant  Value=0  OutDataTypeStr=double  SampleTime=1/44100
  Delay{1..7} (7 alike) : Delay  DelayLength=1  SampleTime=1/44100
  Divide : Product  Inputs=*/  OutDataTypeStr=double
  Gain1 : Gain  Gain=-1  ParamDataTypeStr=fixdt(1,16,12)  OutMin=-1  OutMax=-0.99  OutDataTypeStr=double
  Length : Constant  Value=lambda2*2  OutDataTypeStr=double  SampleTime=1/44100
  Relational Operator1 : RelationalOperator  Operator===  OutDataTypeStr=boolean  RndMeth=Simplest
  Relational Operator2 : RelationalOperator  Operator=>  OutDataTypeStr=boolean  RndMeth=Simplest
  Relational Operator3 : RelationalOperator  Operator=<  OutDataTypeStr=boolean  RndMeth=Simplest
  Relational Operator4 : RelationalOperator  Operator=>  OutDataTypeStr=boolean  RndMeth=Simplest
  Relational Operator5 : RelationalOperator  Operator=<  OutDataTypeStr=boolean  RndMeth=Simplest
  Relational Operator6 : RelationalOperator  Operator=>  OutDataTypeStr=boolean  RndMeth=Simplest
  Relational Operator7 : RelationalOperator  Operator===  OutDataTypeStr=boolean  RndMeth=Simplest
  Subtract1 : Sum  Inputs=+-  AccumDataTypeStr=double  OutDataTypeStr=double
  Threshold_Switch : Switch  Threshold=1  OutDataTypeStr=double
  Threshold_Switch1 : Switch  Threshold=1  OutDataTypeStr=double
  Threshold_Switch2 : Switch  Threshold=1  OutDataTypeStr=double
  New_Threshold : Outport  OutDataTypeStr=double  SampleTime=1/44100
  wires:
  Threshold_Switch/1 -> Threshold_Switch2/3
  Relational Operator6/1 -> Threshold_Switch1/2
  Gain1/1 -> Relational Operator3/2
  Delay4/1 -> Threshold_Switch/3
  Add1/1 -> Delay4/1
  Delay2/1 -> Relational Operator4/1
  Delay3/1 -> Relational Operator4/2
  Delay1/1 -> Threshold_Switch/1
  Relational Operator2/1 -> Delay2/1
  Relational Operator3/1 -> Delay3/1
  Relational Operator5/1 -> Delay6/1
  Delay6/1 -> Relational Operator6/2
  Delay5/1 -> Relational Operator6/1
  Threshold1/1 -> Relational Operator2/2, Subtract1/2, Relational Operator5/2, Relational Operator1/2, Add1/2, Gain1/1, Relational Operator7/2
  Abs/1 -> Relational Operator1/1
  Relational Operator4/1 -> Threshold_Switch/2
  Subtract1/1 -> Delay1/1
  Constant/1 -> Threshold_Switch1/3, Threshold_Switch1/1
  Signal_w/1 -> Subtract1/1, Relational Operator2/1, Relational Operator5/1, Abs/1, Add1/1, Relational Operator3/1, Relational Operator7/1
  Relational Operator7/1 -> Threshold_Switch2/2
  Relational Operator1/1 -> Delay5/1
  Threshold_Switch1/1 -> Threshold_Switch2/1
  Threshold_Switch2/1 -> Divide/1
  Length/1 -> Divide/2
  Divide/1 -> Delay7/1
  Delay7/1 -> New_Threshold/1

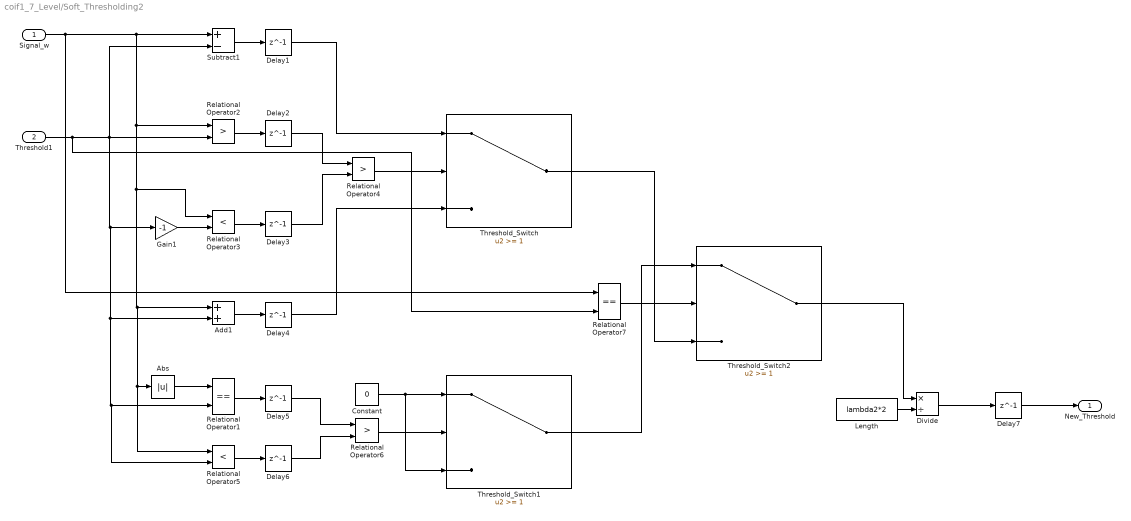
== system coif1_7_Level/Soft_Thresholding2 ==
  Signal_w : Inport  OutDataTypeStr=double  SampleTime=1/44100
  Threshold1 : Inport  Port=2  OutDataTypeStr=double  SampleTime=1/44100
  Abs : Abs  OutDataTypeStr=double
  Add1 : Sum  AccumDataTypeStr=double  OutDataTypeStr=double
  Constant : Constant  Value=0  OutDataTypeStr=double  SampleTime=1/44100
  Delay{1..7} (7 alike) : Delay  DelayLength=1  SampleTime=1/44100
  Divide : Product  Inputs=*/  OutDataTypeStr=double
  Gain1 : Gain  Gain=-1  ParamDataTypeStr=fixdt(1,16,12)  OutMin=-1  OutMax=-0.99  OutDataTypeStr=double
  Length : Constant  Value=lambda2*2  OutDataTypeStr=double  SampleTime=1/44100
  Relational Operator1 : RelationalOperator  Operator===  OutDataTypeStr=boolean  RndMeth=Simplest
  Relational Operator2 : RelationalOperator  Operator=>  OutDataTypeStr=boolean  RndMeth=Simplest
  Relational Operator3 : RelationalOperator  Operator=<  OutDataTypeStr=boolean  RndMeth=Simplest
  Relational Operator4 : RelationalOperator  Operator=>  OutDataTypeStr=boolean  RndMeth=Simplest
  Relational Operator5 : RelationalOperator  Operator=<  OutDataTypeStr=boolean  RndMeth=Simplest
  Relational Operator6 : RelationalOperator  Operator=>  OutDataTypeStr=boolean  RndMeth=Simplest
  Relational Operator7 : RelationalOperator  Operator===  OutDataTypeStr=boolean  RndMeth=Simplest
  Subtract1 : Sum  Inputs=+-  AccumDataTypeStr=double  OutDataTypeStr=double
  Threshold_Switch : Switch  Threshold=1  OutDataTypeStr=double
  Threshold_Switch1 : Switch  Threshold=1  OutDataTypeStr=double
  Threshold_Switch2 : Switch  Threshold=1  OutDataTypeStr=double
  New_Threshold : Outport  OutDataTypeStr=double  SampleTime=1/44100
  wires:
  Threshold_Switch/1 -> Threshold_Switch2/3
  Relational Operator6/1 -> Threshold_Switch1/2
  Gain1/1 -> Relational Operator3/2
  Delay4/1 -> Threshold_Switch/3
  Add1/1 -> Delay4/1
  Delay2/1 -> Relational Operator4/1
  Delay3/1 -> Relational Operator4/2
  Delay1/1 -> Threshold_Switch/1
  Relational Operator2/1 -> Delay2/1
  Relational Operator3/1 -> Delay3/1
  Relational Operator5/1 -> Delay6/1
  Delay6/1 -> Relational Operator6/2
  Delay5/1 -> Relational Operator6/1
  Threshold1/1 -> Relational Operator2/2, Subtract1/2, Relational Operator5/2, Relational Operator1/2, Add1/2, Gain1/1, Relational Operator7/2
  Abs/1 -> Relational Operator1/1
  Relational Operator4/1 -> Threshold_Switch/2
  Subtract1/1 -> Delay1/1
  Constant/1 -> Threshold_Switch1/3, Threshold_Switch1/1
  Signal_w/1 -> Subtract1/1, Relational Operator2/1, Relational Operator5/1, Abs/1, Add1/1, Relational Operator3/1, Relational Operator7/1
  Relational Operator7/1 -> Threshold_Switch2/2
  Relational Operator1/1 -> Delay5/1
  Threshold_Switch1/1 -> Threshold_Switch2/1
  Threshold_Switch2/1 -> Divide/1
  Length/1 -> Divide/2
  Divide/1 -> Delay7/1
  Delay7/1 -> New_Threshold/1

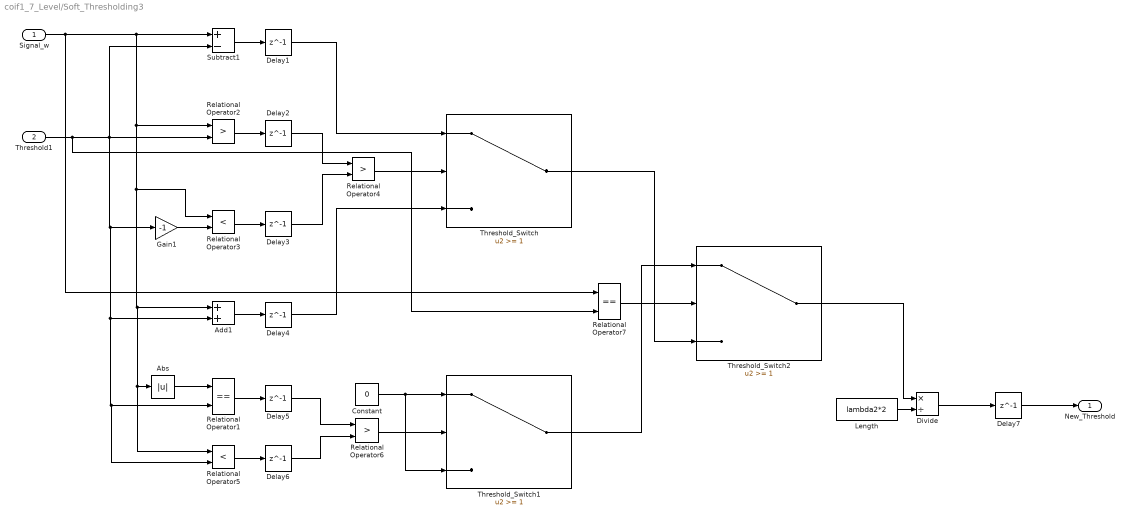
== system coif1_7_Level/Soft_Thresholding3 ==
  Signal_w : Inport  OutDataTypeStr=double  SampleTime=1/44100
  Threshold1 : Inport  Port=2  OutDataTypeStr=double  SampleTime=1/44100
  Abs : Abs  OutDataTypeStr=double
  Add1 : Sum  AccumDataTypeStr=double  OutDataTypeStr=double
  Constant : Constant  Value=0  OutDataTypeStr=double  SampleTime=1/44100
  Delay{1..7} (7 alike) : Delay  DelayLength=1  SampleTime=1/44100
  Divide : Product  Inputs=*/  OutDataTypeStr=double
  Gain1 : Gain  Gain=-1  ParamDataTypeStr=fixdt(1,16,12)  OutMin=-1  OutMax=-0.99  OutDataTypeStr=double
  Length : Constant  Value=lambda2*2  OutDataTypeStr=double  SampleTime=1/44100
  Relational Operator1 : RelationalOperator  Operator===  OutDataTypeStr=boolean  RndMeth=Simplest
  Relational Operator2 : RelationalOperator  Operator=>  OutDataTypeStr=boolean  RndMeth=Simplest
  Relational Operator3 : RelationalOperator  Operator=<  OutDataTypeStr=boolean  RndMeth=Simplest
  Relational Operator4 : RelationalOperator  Operator=>  OutDataTypeStr=boolean  RndMeth=Simplest
  Relational Operator5 : RelationalOperator  Operator=<  OutDataTypeStr=boolean  RndMeth=Simplest
  Relational Operator6 : RelationalOperator  Operator=>  OutDataTypeStr=boolean  RndMeth=Simplest
  Relational Operator7 : RelationalOperator  Operator===  OutDataTypeStr=boolean  RndMeth=Simplest
  Subtract1 : Sum  Inputs=+-  AccumDataTypeStr=double  OutDataTypeStr=double
  Threshold_Switch : Switch  Threshold=1  OutDataTypeStr=double
  Threshold_Switch1 : Switch  Threshold=1  OutDataTypeStr=double
  Threshold_Switch2 : Switch  Threshold=1  OutDataTypeStr=double
  New_Threshold : Outport  OutDataTypeStr=double  SampleTime=1/44100
  wires:
  Threshold_Switch/1 -> Threshold_Switch2/3
  Relational Operator6/1 -> Threshold_Switch1/2
  Gain1/1 -> Relational Operator3/2
  Delay4/1 -> Threshold_Switch/3
  Add1/1 -> Delay4/1
  Delay2/1 -> Relational Operator4/1
  Delay3/1 -> Relational Operator4/2
  Delay1/1 -> Threshold_Switch/1
  Relational Operator2/1 -> Delay2/1
  Relational Operator3/1 -> Delay3/1
  Relational Operator5/1 -> Delay6/1
  Delay6/1 -> Relational Operator6/2
  Delay5/1 -> Relational Operator6/1
  Threshold1/1 -> Relational Operator2/2, Subtract1/2, Relational Operator5/2, Relational Operator1/2, Add1/2, Gain1/1, Relational Operator7/2
  Abs/1 -> Relational Operator1/1
  Relational Operator4/1 -> Threshold_Switch/2
  Subtract1/1 -> Delay1/1
  Constant/1 -> Threshold_Switch1/3, Threshold_Switch1/1
  Signal_w/1 -> Subtract1/1, Relational Operator2/1, Relational Operator5/1, Abs/1, Add1/1, Relational Operator3/1, Relational Operator7/1
  Relational Operator7/1 -> Threshold_Switch2/2
  Relational Operator1/1 -> Delay5/1
  Threshold_Switch1/1 -> Threshold_Switch2/1
  Threshold_Switch2/1 -> Divide/1
  Length/1 -> Divide/2
  Divide/1 -> Delay7/1
  Delay7/1 -> New_Threshold/1

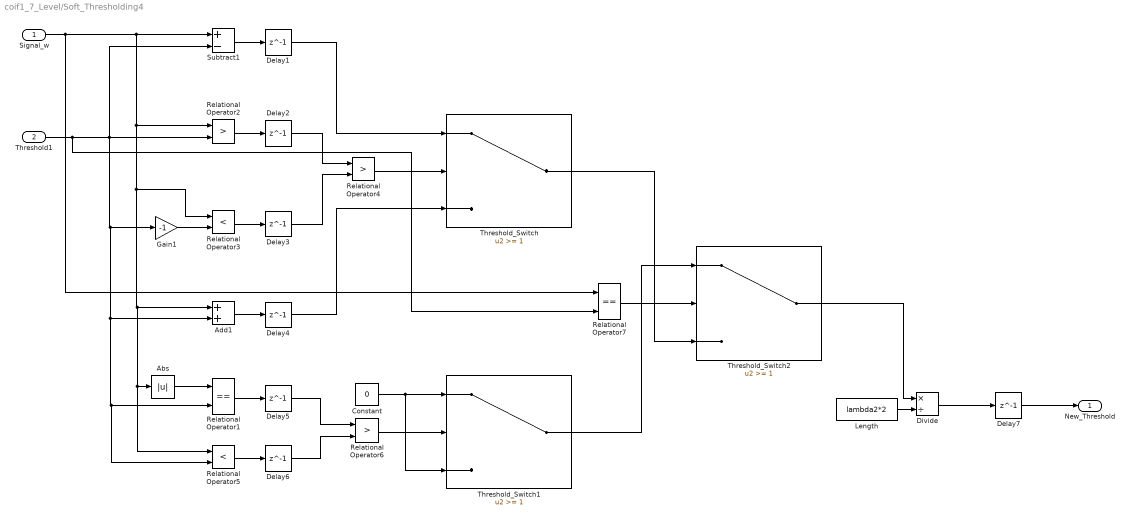
== system coif1_7_Level/Soft_Thresholding4 ==
  Signal_w : Inport  OutDataTypeStr=double  SampleTime=1/44100
  Threshold1 : Inport  Port=2  OutDataTypeStr=double  SampleTime=1/44100
  Abs : Abs  OutDataTypeStr=double
  Add1 : Sum  AccumDataTypeStr=double  OutDataTypeStr=double
  Constant : Constant  Value=0  OutDataTypeStr=double  SampleTime=1/44100
  Delay{1..7} (7 alike) : Delay  DelayLength=1  SampleTime=1/44100
  Divide : Product  Inputs=*/  OutDataTypeStr=double
  Gain1 : Gain  Gain=-1  ParamDataTypeStr=fixdt(1,16,12)  OutMin=-1  OutMax=-0.99  OutDataTypeStr=double
  Length : Constant  Value=lambda2*2  OutDataTypeStr=double  SampleTime=1/44100
  Relational Operator1 : RelationalOperator  Operator===  OutDataTypeStr=boolean  RndMeth=Simplest
  Relational Operator2 : RelationalOperator  Operator=>  OutDataTypeStr=boolean  RndMeth=Simplest
  Relational Operator3 : RelationalOperator  Operator=<  OutDataTypeStr=boolean  RndMeth=Simplest
  Relational Operator4 : RelationalOperator  Operator=>  OutDataTypeStr=boolean  RndMeth=Simplest
  Relational Operator5 : RelationalOperator  Operator=<  OutDataTypeStr=boolean  RndMeth=Simplest
  Relational Operator6 : RelationalOperator  Operator=>  OutDataTypeStr=boolean  RndMeth=Simplest
  Relational Operator7 : RelationalOperator  Operator===  OutDataTypeStr=boolean  RndMeth=Simplest
  Subtract1 : Sum  Inputs=+-  AccumDataTypeStr=double  OutDataTypeStr=double
  Threshold_Switch : Switch  Threshold=1  OutDataTypeStr=double
  Threshold_Switch1 : Switch  Threshold=1  OutDataTypeStr=double
  Threshold_Switch2 : Switch  Threshold=1  OutDataTypeStr=double
  New_Threshold : Outport  OutDataTypeStr=double  SampleTime=1/44100
  wires:
  Threshold_Switch/1 -> Threshold_Switch2/3
  Relational Operator6/1 -> Threshold_Switch1/2
  Gain1/1 -> Relational Operator3/2
  Delay4/1 -> Threshold_Switch/3
  Add1/1 -> Delay4/1
  Delay2/1 -> Relational Operator4/1
  Delay3/1 -> Relational Operator4/2
  Delay1/1 -> Threshold_Switch/1
  Relational Operator2/1 -> Delay2/1
  Relational Operator3/1 -> Delay3/1
  Relational Operator5/1 -> Delay6/1
  Delay6/1 -> Relational Operator6/2
  Delay5/1 -> Relational Operator6/1
  Threshold1/1 -> Relational Operator2/2, Subtract1/2, Relational Operator5/2, Relational Operator1/2, Add1/2, Gain1/1, Relational Operator7/2
  Abs/1 -> Relational Operator1/1
  Relational Operator4/1 -> Threshold_Switch/2
  Subtract1/1 -> Delay1/1
  Constant/1 -> Threshold_Switch1/3, Threshold_Switch1/1
  Signal_w/1 -> Subtract1/1, Relational Operator2/1, Relational Operator5/1, Abs/1, Add1/1, Relational Operator3/1, Relational Operator7/1
  Relational Operator7/1 -> Threshold_Switch2/2
  Relational Operator1/1 -> Delay5/1
  Threshold_Switch1/1 -> Threshold_Switch2/1
  Threshold_Switch2/1 -> Divide/1
  Length/1 -> Divide/2
  Divide/1 -> Delay7/1
  Delay7/1 -> New_Threshold/1

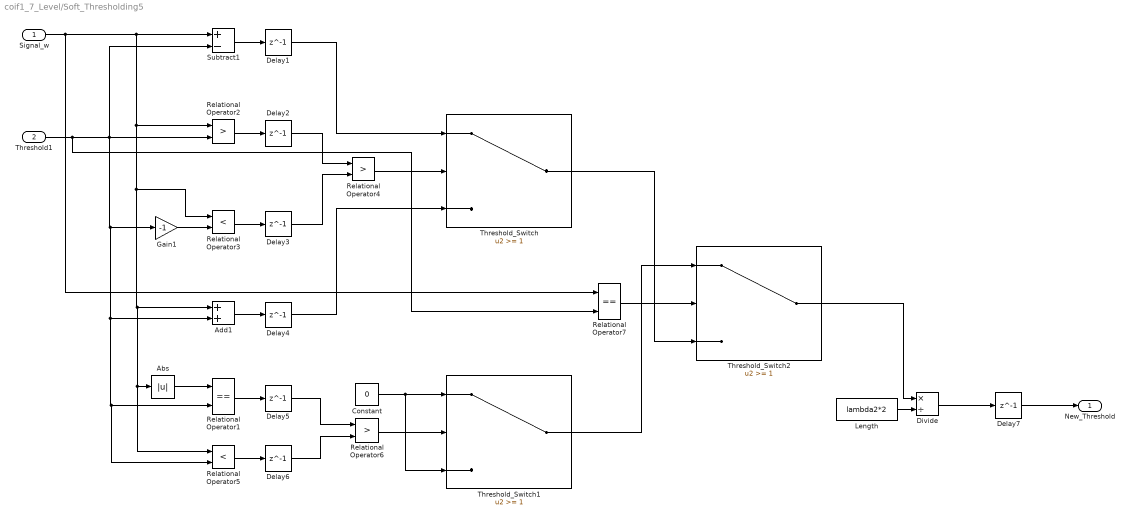
== system coif1_7_Level/Soft_Thresholding5 ==
  Signal_w : Inport  OutDataTypeStr=double  SampleTime=1/44100
  Threshold1 : Inport  Port=2  OutDataTypeStr=double  SampleTime=1/44100
  Abs : Abs  OutDataTypeStr=double
  Add1 : Sum  AccumDataTypeStr=double  OutDataTypeStr=double
  Constant : Constant  Value=0  OutDataTypeStr=double  SampleTime=1/44100
  Delay{1..7} (7 alike) : Delay  DelayLength=1  SampleTime=1/44100
  Divide : Product  Inputs=*/  OutDataTypeStr=double
  Gain1 : Gain  Gain=-1  ParamDataTypeStr=fixdt(1,16,12)  OutMin=-1  OutMax=-0.99  OutDataTypeStr=double
  Length : Constant  Value=lambda2*2  OutDataTypeStr=double  SampleTime=1/44100
  Relational Operator1 : RelationalOperator  Operator===  OutDataTypeStr=boolean  RndMeth=Simplest
  Relational Operator2 : RelationalOperator  Operator=>  OutDataTypeStr=boolean  RndMeth=Simplest
  Relational Operator3 : RelationalOperator  Operator=<  OutDataTypeStr=boolean  RndMeth=Simplest
  Relational Operator4 : RelationalOperator  Operator=>  OutDataTypeStr=boolean  RndMeth=Simplest
  Relational Operator5 : RelationalOperator  Operator=<  OutDataTypeStr=boolean  RndMeth=Simplest
  Relational Operator6 : RelationalOperator  Operator=>  OutDataTypeStr=boolean  RndMeth=Simplest
  Relational Operator7 : RelationalOperator  Operator===  OutDataTypeStr=boolean  RndMeth=Simplest
  Subtract1 : Sum  Inputs=+-  AccumDataTypeStr=double  OutDataTypeStr=double
  Threshold_Switch : Switch  Threshold=1  OutDataTypeStr=double
  Threshold_Switch1 : Switch  Threshold=1  OutDataTypeStr=double
  Threshold_Switch2 : Switch  Threshold=1  OutDataTypeStr=double
  New_Threshold : Outport  OutDataTypeStr=double  SampleTime=1/44100
  wires:
  Threshold_Switch/1 -> Threshold_Switch2/3
  Relational Operator6/1 -> Threshold_Switch1/2
  Gain1/1 -> Relational Operator3/2
  Delay4/1 -> Threshold_Switch/3
  Add1/1 -> Delay4/1
  Delay2/1 -> Relational Operator4/1
  Delay3/1 -> Relational Operator4/2
  Delay1/1 -> Threshold_Switch/1
  Relational Operator2/1 -> Delay2/1
  Relational Operator3/1 -> Delay3/1
  Relational Operator5/1 -> Delay6/1
  Delay6/1 -> Relational Operator6/2
  Delay5/1 -> Relational Operator6/1
  Threshold1/1 -> Relational Operator2/2, Subtract1/2, Relational Operator5/2, Relational Operator1/2, Add1/2, Gain1/1, Relational Operator7/2
  Abs/1 -> Relational Operator1/1
  Relational Operator4/1 -> Threshold_Switch/2
  Subtract1/1 -> Delay1/1
  Constant/1 -> Threshold_Switch1/3, Threshold_Switch1/1
  Signal_w/1 -> Subtract1/1, Relational Operator2/1, Relational Operator5/1, Abs/1, Add1/1, Relational Operator3/1, Relational Operator7/1
  Relational Operator7/1 -> Threshold_Switch2/2
  Relational Operator1/1 -> Delay5/1
  Threshold_Switch1/1 -> Threshold_Switch2/1
  Threshold_Switch2/1 -> Divide/1
  Length/1 -> Divide/2
  Divide/1 -> Delay7/1
  Delay7/1 -> New_Threshold/1

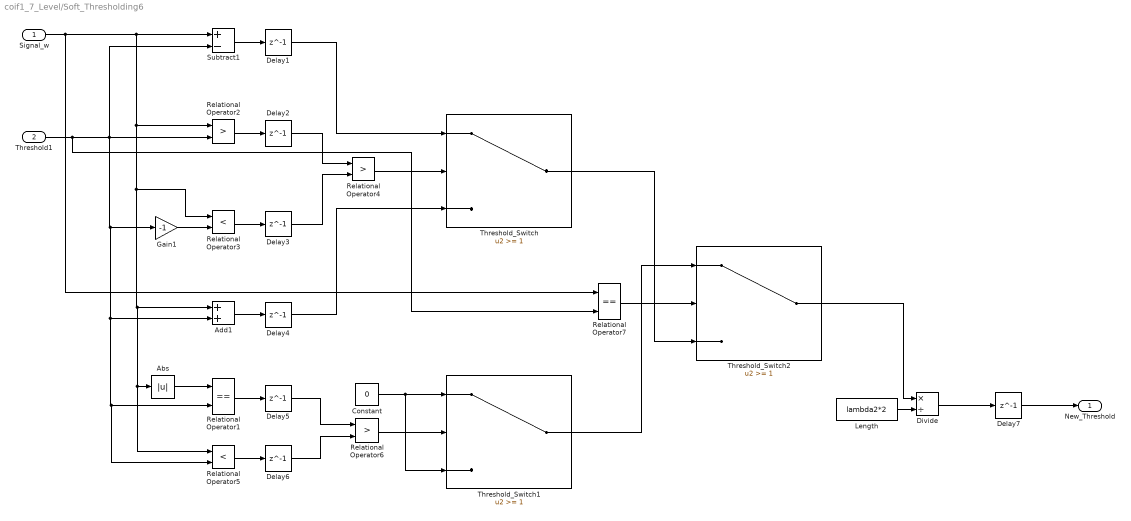
== system coif1_7_Level/Soft_Thresholding6 ==
  Signal_w : Inport  OutDataTypeStr=double  SampleTime=1/44100
  Threshold1 : Inport  Port=2  OutDataTypeStr=double  SampleTime=1/44100
  Abs : Abs  OutDataTypeStr=double
  Add1 : Sum  AccumDataTypeStr=double  OutDataTypeStr=double
  Constant : Constant  Value=0  OutDataTypeStr=double  SampleTime=1/44100
  Delay{1..7} (7 alike) : Delay  DelayLength=1  SampleTime=1/44100
  Divide : Product  Inputs=*/  OutDataTypeStr=double
  Gain1 : Gain  Gain=-1  ParamDataTypeStr=fixdt(1,16,12)  OutMin=-1  OutMax=-0.99  OutDataTypeStr=double
  Length : Constant  Value=lambda2*2  OutDataTypeStr=double  SampleTime=1/44100
  Relational Operator1 : RelationalOperator  Operator===  OutDataTypeStr=boolean  RndMeth=Simplest
  Relational Operator2 : RelationalOperator  Operator=>  OutDataTypeStr=boolean  RndMeth=Simplest
  Relational Operator3 : RelationalOperator  Operator=<  OutDataTypeStr=boolean  RndMeth=Simplest
  Relational Operator4 : RelationalOperator  Operator=>  OutDataTypeStr=boolean  RndMeth=Simplest
  Relational Operator5 : RelationalOperator  Operator=<  OutDataTypeStr=boolean  RndMeth=Simplest
  Relational Operator6 : RelationalOperator  Operator=>  OutDataTypeStr=boolean  RndMeth=Simplest
  Relational Operator7 : RelationalOperator  Operator===  OutDataTypeStr=boolean  RndMeth=Simplest
  Subtract1 : Sum  Inputs=+-  AccumDataTypeStr=double  OutDataTypeStr=double
  Threshold_Switch : Switch  Threshold=1  OutDataTypeStr=double
  Threshold_Switch1 : Switch  Threshold=1  OutDataTypeStr=double
  Threshold_Switch2 : Switch  Threshold=1  OutDataTypeStr=double
  New_Threshold : Outport  OutDataTypeStr=double  SampleTime=1/44100
  wires:
  Threshold_Switch/1 -> Threshold_Switch2/3
  Relational Operator6/1 -> Threshold_Switch1/2
  Gain1/1 -> Relational Operator3/2
  Delay4/1 -> Threshold_Switch/3
  Add1/1 -> Delay4/1
  Delay2/1 -> Relational Operator4/1
  Delay3/1 -> Relational Operator4/2
  Delay1/1 -> Threshold_Switch/1
  Relational Operator2/1 -> Delay2/1
  Relational Operator3/1 -> Delay3/1
  Relational Operator5/1 -> Delay6/1
  Delay6/1 -> Relational Operator6/2
  Delay5/1 -> Relational Operator6/1
  Threshold1/1 -> Relational Operator2/2, Subtract1/2, Relational Operator5/2, Relational Operator1/2, Add1/2, Gain1/1, Relational Operator7/2
  Abs/1 -> Relational Operator1/1
  Relational Operator4/1 -> Threshold_Switch/2
  Subtract1/1 -> Delay1/1
  Constant/1 -> Threshold_Switch1/3, Threshold_Switch1/1
  Signal_w/1 -> Subtract1/1, Relational Operator2/1, Relational Operator5/1, Abs/1, Add1/1, Relational Operator3/1, Relational Operator7/1
  Relational Operator7/1 -> Threshold_Switch2/2
  Relational Operator1/1 -> Delay5/1
  Threshold_Switch1/1 -> Threshold_Switch2/1
  Threshold_Switch2/1 -> Divide/1
  Length/1 -> Divide/2
  Divide/1 -> Delay7/1
  Delay7/1 -> New_Threshold/1

== system coif1_7_Level/Threshold_Estimator ==
  Signal_w : Inport  OutDataTypeStr=double  SampleTime=1/44100
  Absolute_Value1 : Subsystem
  Length : Constant  Value=lambda2  OutDataTypeStr=double  SampleTime=1/44100
  Median2 : Subsystem
  Multiply : Product  OutDataTypeStr=double
  Threshold : Outport  OutDataTypeStr=double  SampleTime=1/44100  VectorParamsAs1DForOutWhenUnconnected=off
  wires:
  Length/1 -> Multiply/2
  Median2/1(Median) -> Multiply/1
  Absolute_Value1/1(Out_Abs) -> Median2/1(Signal_w3)
  Signal_w/1 -> Absolute_Value1/1(Signal_w4)
  Multiply/1 -> Threshold/1
